simulink model "cw2sim"  (R2022b)
settings: Solver=ode23tb  StartTime=0.0  StopTime=100e-3  MaxStep=Ts  RelTol=1e-3
values from neighbouring files (symbols this model uses):
  C = 1e-3    (= 0.001)    [Parametry_DCDC.m]
  L = 1e-3    (= 0.001)    [Parametry_DCDC.m]
  RAMP_on = 1    [Parametry_DCDC.m]
  RL = 50e-3    (= 0.05)    [Parametry_DCDC.m]
  Rload = 10    [Parametry_DCDC.m]
  Ts = (1/fsw)/1000    (= 5e-08)    [Parametry_DCDC.m]
  Uin = 100    [Parametry_DCDC.m]
undefined symbols (not defined in the file or in its folder): sigbuilder_block
libraries: spsSeriesRLCBranchLib x3, spsGroundLib x2, spsCurrentMeasurementLib x1, spsDCVoltageSourceLib x1, spsDiodeLib x1, spsIGBTDiodeLib x1, simulink x1, spsVoltageMeasurementLib x1, sps_lib x1
settings Model: Creator=Acer  LastModifiedBy=Acer
settings DataIOCC: ReturnWorkspaceOutputs=off

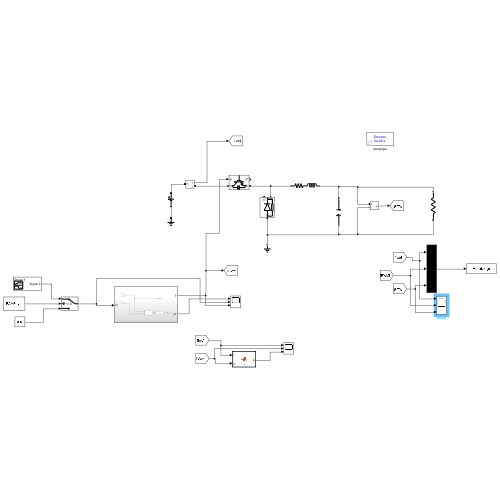
[thumbnail: Simulink's stored preview of the top-level diagram]
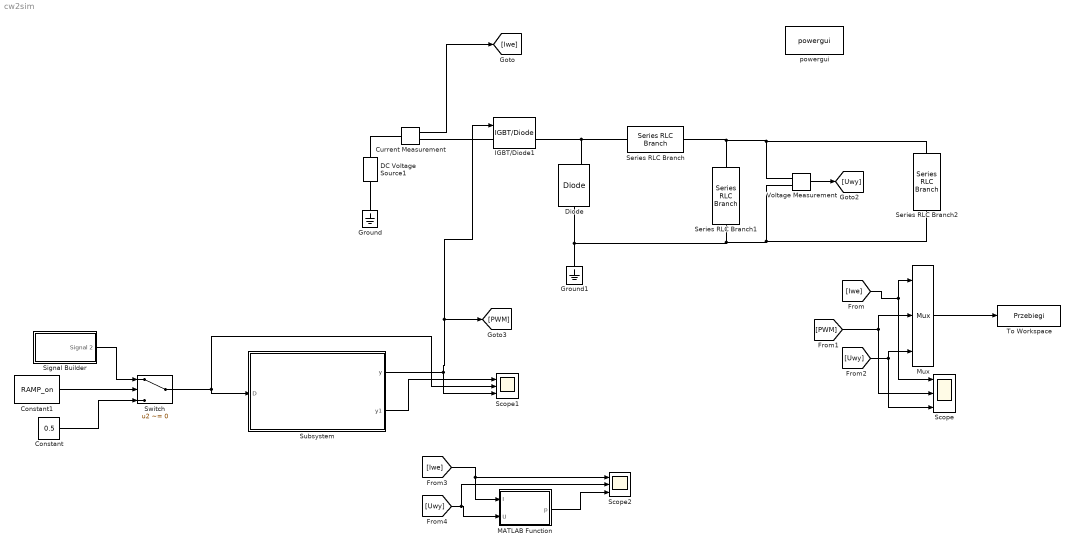
== system cw2sim ==
  Constant : Constant  Value=0.5
  Constant1 : Constant  Value=RAMP_on
  Current Measurement : spsCurrentMeasurementLib/Current Measurement  PhasorSimulation=off  OutputType=Complex  PSBequivalent=0
  DC Voltage Source1 : spsDCVoltageSourceLib/DC Voltage Source  Amplitude=Uin  Measurements=None
  Diode : spsDiodeLib/Diode  Ron=0.001  Lon=0  Vf=0.8  IC=0  UseSnubber=0  Rs=500  Cs=250e-9  Measurements=on
  Ground : spsGroundLib/Ground  LConnTagsString=a
  Ground1 : spsGroundLib/Ground  LConnTagsString=a
  IGBT/Diode1 : spsIGBTDiodeLib/IGBT//Diode  Ron=Rdson  Rs=1e5  Cs=inf  Measurements=on
  MATLAB Function : MATLAB Function  TreatAsAtomicUnit=on
  Mux : Mux  Inputs=3
  Scope : Scope  NumInputPorts=3
  Scope1 : Scope  NumInputPorts=3
  Scope2 : Scope  NumInputPorts=3
  Series RLC Branch : spsSeriesRLCBranchLib/Series RLC Branch  LConnTagsString=__new0  RConnTagsString=__new0  BranchType=RL  Resistance=RL  Inductance=L  SetiL0=off  InitialCurrent=0  Capacitance=1e-6  Setx0=off  InitialVoltage=0  Measurements=None
  Series RLC Branch1 : spsSeriesRLCBranchLib/Series RLC Branch  LConnTagsString=__new0  RConnTagsString=__new0  BranchType=C  Resistance=1  Inductance=1e-3  SetiL0=off  InitialCurrent=0  Capacitance=C  Setx0=off  InitialVoltage=0  Measurements=None
  Series RLC Branch2 : spsSeriesRLCBranchLib/Series RLC Branch  LConnTagsString=__new0  RConnTagsString=__new0  BranchType=R  Resistance=Rload  Inductance=1e-3  SetiL0=off  InitialCurrent=0  Capacitance=1e-6  Setx0=off  InitialVoltage=0  Measurements=None
  Signal Builder : Subsystem  Tag=STV Subsys  LoadFcn=sigbuilder_block('load');  StartFcn=sigbuilder_block('start');  StopFcn=sigbuilder_block('stop');  ClipboardFcn=sigbuilder_block('clipboard');  mask(Sigbuilder block){tuvar=[0:10]}
      mask help: Simulink:masks:SigbuilderBlock_MD
      mask init:
      | if ~strcmp(get_param(bdroot(gcbh),'SimulationStatus'),'stopped') tuvar = sigbuilder_block('maskInit'); end
      settings: CopyFcn=sigbuilder_block('copy');  DeleteFcn=sigbuilder_block('delete');  ModelCloseFcn=sigbuilder_block('modelClose');  PreSaveFcn=sigbuilder_block('preSave');  PauseFcn=sigbuilder_block('pause');  ContinueFcn=sigbuilder_block('continue');  NameChangeFcn=sigbuilder_block('namechange');  OpenFcn=sigbuilder_block('open',[313.2 19.8 550.8 400.2 ]);  CloseFcn=sigbuilder_block('close');
      mask Display: plot(0, 0, 100, 100,[2, 2, 32, 32, 2], [68, 8, 8, 68, 68],[32, 2], [38, 38], [32, 19, 2],[53, 60, 44], [32, 17, 17, 2],[16, 16, 31, 31]);txt = getActiveGroup(gcbh);text(2, 100, txt,'verticalAlignment', 'top');
  Subsystem : Subsystem
  Switch : Switch  Criteria=u2 ~= 0  SaturateOnIntegerOverflow=off  InputSameDT=off
  To Workspace : ToWorkspace  VariableName=Przebiegi  SaveFormat=Structure With Time  SampleTime=-1
  Voltage Measurement : spsVoltageMeasurementLib/Voltage Measurement  PhasorSimulation=off  OutputType=Complex  PSBequivalent=0
  powergui : sps_lib/powergui  Priority=1  SimulationMode=Discrete  SampleTime=Ts/4  frequency=60  Iterations=50  frequencyindice=0  Pbase=100e6  ErrMax=1e-4  UnitsV=kV  UnitsW=MW  buscounter=0  FunctionMessages=off  echomessages=off  EnableUseOfTLC=off  CurrentSourceSwitches=off  DisableSnubberDevices=off  DisableRonSwitches=off  DisableVfSwitches=off  DisplayEquations=off  AutomaticDiscreteSolvers=off  SolverType=Tustin/Backward Euler (TBE)  Interpol=off  ExternalGateDelay=off  methode=off  Ts=100  x0status=blocks  SPID=on  SwTol=0  HookPort=off  NonlinearTolerance=1e-4  nMaxIteration=100  ContinueOnMaxIteration=off  RestoreLinks=warning  ResistiveCurrentMeasurement=off  Frange=[0:2:500]  Ylog=off  Xlog=on  ShowGrid=off  save=off  variable=ZData  structure=0  ZoomFFT=off  StartTime=0.0  cycles=1  DisplayStyle=1  fundamental=60  FreqAxis=off  MaxFrequency=1000  frequencyindicesteady=1  RmsSteady=1  display=off
  wires:
  Current Measurement/1 -> [Iwe]
  Voltage Measurement/1 -> [Uwy]
  [Iwe] -> Scope/1, Mux/1
  [PWM] -> Scope/2, Mux/2
  [Uwy] -> Scope/3, Mux/3
  Mux/1 -> To Workspace/1
  Subsystem/1(y) -> Scope1/3, IGBT/Diode1/1, [PWM]
  Switch/1 -> Subsystem/1(D), Scope1/2
  Signal Builder/1(Signal 2) -> Switch/1
  Constant1/1 -> Switch/2
  Constant/1 -> Switch/3
  MATLAB Function/1(p) -> Scope2/3
  [Iwe] -> Scope2/1, MATLAB Function/1(I)
  [Uwy] -> Scope2/2, MATLAB Function/2(U)
  Subsystem/2(y1) -> Scope1/1
  connections:
  Ground/LConn1 -- DC Voltage Source1/LConn1
  DC Voltage Source1/RConn1 -- Current Measurement/LConn1
  IGBT/Diode1/LConn1 -- Current Measurement/RConn1
  Series RLC Branch/LConn1 -- IGBT/Diode1/RConn1 -- Diode/RConn1
  Ground1/LConn1 -- Series RLC Branch2/RConn1 -- Voltage Measurement/LConn2 -- Series RLC Branch1/RConn1 -- Diode/LConn1
  Series RLC Branch1/LConn1 -- Series RLC Branch2/LConn1 -- Voltage Measurement/LConn1 -- Series RLC Branch/RConn1

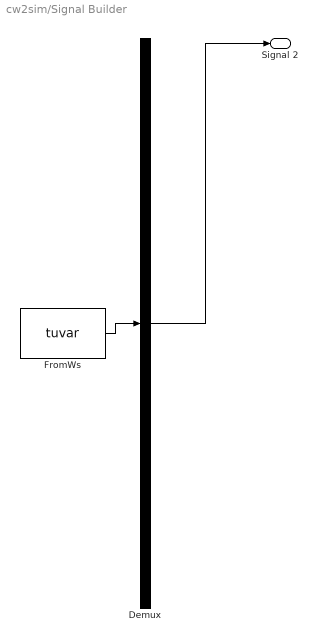
== system cw2sim/Signal Builder ==
  Demux : Demux  Tag=STV Demux  Outputs=1
      settings: DisplayOption=none
  FromWs : FromWorkspace  Tag=STV FromWs  VariableName=tuvar
      SigBuilderData=|
      | common.afterFinalStr = 'Extrapolate'
      | common.sampleTime = 0
      | dataSet.timeRange = [0 0.2]
      | dataSet.name = 'Group 1'
      | sbobj.Groups.Name = 'Group 1'
      | sbobj.Groups.Signals.Name = 'Signal 2'
      | sbobj.Groups.Signals.XData = [0 0.01 0.2]
      | sbobj.Groups.Signals.YData = [0 0.5 0.5]
      | sbobj.Groups.TimeRange = [0 0.2]
  Signal 2 : Outport  Tag=STV Outport
  wires:
  Demux/1 -> Signal 2/1
  FromWs/1 -> Demux/1

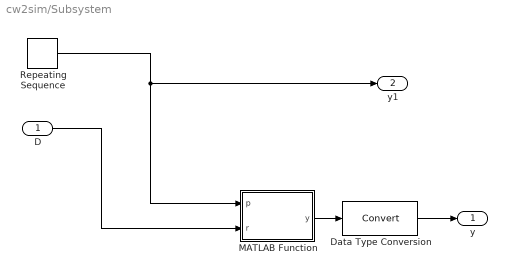
== system cw2sim/Subsystem ==
  D : Inport
  Data Type Conversion : DataTypeConversion  SaturateOnIntegerOverflow=off  RndMeth=Floor
  MATLAB Function : MATLAB Function  TreatAsAtomicUnit=on
  Repeating Sequence : simulink/Sources/Repeating Sequence  rep_seq_t=[0 50e-6]  rep_seq_y=[0 1]
  y : Outport
  y1 : Outport  Port=2
  wires:
  Repeating Sequence/1 -> y1/1, MATLAB Function/1(p)
  D/1 -> MATLAB Function/2(r)
  MATLAB Function/1(y) -> Data Type Conversion/1
  Data Type Conversion/1 -> y/1

== matlab function cw2sim/MATLAB Function ==
  data: I input; p output; U input
function p = fcn(I,U)

p =U*I;

== matlab function cw2sim/Subsystem/MATLAB Function ==
  data: p input; y output; r input
function y = fcn(p,r)

z = p-r;
if z<=0
    y=1;
else
    y=0;
end
